simulink model "doc_noisevariance_ebno"  (R2014a)
settings: Solver=FixedStepDiscrete  SolverMode=SingleTasking  StartTime=0.0  StopTime=inf  RelTol=1e-3
PreLoadFcn:
  | Ts = 1e-3; % Sample time
  | EibNo = 4; % EbNo of information bits in dB
  | codeRate = 1/2; % from Trellis structure
  | EbNo = EibNo - 10*log10(1/codeRate); %EbNo of coded bits in dB
  | Pi = 1; % input signal power in watts
libraries: commdigbbndpm3 x2, commcnvcod2 x2, commchan3 x1, commrandsrc2 x1, commsink2 x1, simulink x1
settings Model: RequirementInfo=9  CovMetricSettings=d  ExtModeTrigMode=oneshot  ExtModeArmWhenConnect=off  ExtModeAutoUpdateStatusClock=off  Creator=The MathWorks Inc.
settings DataIOCC: LimitDataPoints=off  SaveFormat=Structure  SignalLoggingSaveFormat=ModelDataLogs  SaveOutput=off  SaveTime=off
settings OptimizationCC: BlockReduction=off  BooleanDataType=off  ExpressionDepthLimit=2147483647  InitFltsAndDblsToZero=on
settings DebuggingCC: SaveWithParameterizedLinksMsg=none  UnderspecifiedInitializationDetection=Classic  SignalResolutionControl=TryResolveAllWithWarning  SolverPrmCheckMsg=none  MultiTaskDSMMsg=warning  MultiTaskCondExecSysMsg=none  SigSpecEnsureSampleTimeMsg=none  IntegerOverflowMsg=none  FcnCallInpInsideContextMsg=UseLocalSettings  StateNameClashWarn=warning  StrictBusMsg=None
settings HardwareCC: TargetUnknown=on
settings RTWCC: IncludeERTFirstTime=on
settings GRTTargetCC: TargetFcnLib=ansi_tfl_tmw.mat  CombineOutputUpdateFcns=off  GRTInterface=on

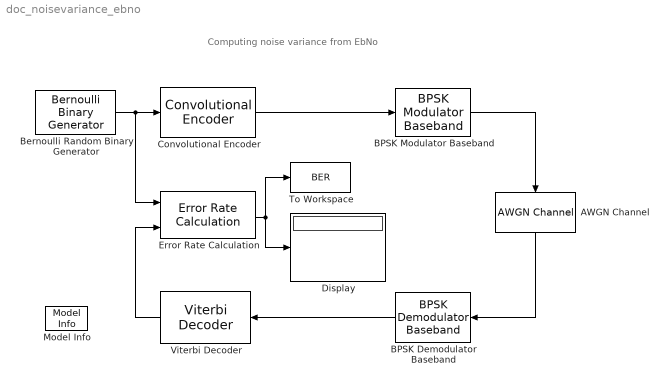
== system doc_noisevariance_ebno ==
  note: Computing noise variance from EbNo
  AWGN Channel : commchan3/AWGN Channel  InputProcessing=Columns as channels (frame based)  seed=1237  noiseMode="Signal to noise ratio  (Eb/No)"  EbNodB=EbNo  EsNodB=-1  SNRdB=10  bitsPerSym=1  Ps=Pi  Tsym=codeRate * Ts  variance=1
  BPSK Demodulator Baseband : commdigbbndpm3/BPSK Demodulator Baseband  Ph=0  DecType=Log-likelihood ratio  VarSource=Dialog  Variance=Pi/(10^(EbNo/10))  outDtype=double  derotateFactorWordLen=16
  BPSK Modulator Baseband : commdigbbndpm3/BPSK Modulator Baseband  Ph=0  outDtype=double  outWordLen=16  outUDDataType=sfix(16)  outFracLenMode=Best precision  outFracLen=15
  Bernoulli Random Binary Generator : commrandsrc2/Bernoulli Binary Generator  P=0.5  seed=25741  Ts=Ts  frameBased=on  sampPerFrame=1e3  orient=off  outDataType=double
  Convolutional Encoder : commcnvcod2/Convolutional Encoder  trellis=poly2trellis(7, [171 133])  opMode=Continuous  DelayedResetAction=off  hasIniStPort=off  hasFinStPort=off  usePuncVector=off  punctureVector=[1; 1; 0; 1; 0; 1]  reset=Unused parameter value
  Display : Display
  Error Rate Calculation : commsink2/Error Rate Calculation  N=48  st_delay=0  cp_mode=Entire frame  subframe=[]  PMode=Port  WsName=ErrorVec  RsMode2=off  stop=on  numErr=100  maxBits=1e7
  Model Info : simulink/Model-Wide Utilities/Model Info  InitialBlockCM=None  BlockCM=none  Frame=on  DisplayStringWithTags=Info  HorizontalTextAlignment=Center  LeftAlignmentValue=0.5  SourceBlockDiagram=doc_noisevariance_ebno  TagMaxNumber=20
  To Workspace : ToWorkspace  VariableName=BER  SampleTime=-1
      settings: MaxDataPoints=1
  Viterbi Decoder : commcnvcod2/Viterbi Decoder  trellis=poly2trellis(7, [171 133])  isPunctured=off  punctureVector=[1; 1; 0; 1; 0; 1]  erasures=off  dectype=Unquantized  runSigValErrCheck=off  nsdecb=3  smWordLength=16  tbdepth=48  opmode=Continuous  reset=off  outDataType=double  delayedResetAction=off
  wires:
  Convolutional Encoder/1 -> BPSK Modulator Baseband/1
  BPSK Modulator Baseband/1 -> AWGN Channel/1
  Bernoulli Random Binary Generator/1 -> Convolutional Encoder/1, Error Rate Calculation/1
  Error Rate Calculation/1 -> Display/1, To Workspace/1
  Viterbi Decoder/1 -> Error Rate Calculation/2
  AWGN Channel/1 -> BPSK Demodulator Baseband/1
  BPSK Demodulator Baseband/1 -> Viterbi Decoder/1
